simulink library "GoodWe_lib"  (Simulink 3.00)
libraries: mathlib x2, inoutlib x1
settings Model: MaskType=REX sequence  MaskIconFrame=on  MaskIconOpaque=on  MaskIconRotate=none  MaskIconUnits=autoscale

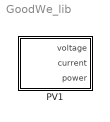
== system GoodWe_lib ==
  PV1 : Subsystem  mask(REX sequence){id=1}
      mask prompts: id "String ID"

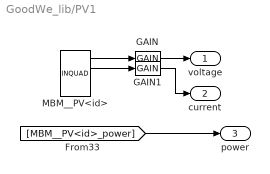
== system GoodWe_lib/PV1 ==
  GAIN : mathlib/GAIN  k=0.1
  GAIN1 : mathlib/GAIN  k=0.1
  MBM__PV<id> : inoutlib/INQUAD
  voltage : Outport  Port=1  OutDataTypeStr=Inherit: auto
  current : Outport  Port=2  OutDataTypeStr=Inherit: auto
  power : Outport  Port=3  OutDataTypeStr=Inherit: auto
  wires:
  [MBM__PV<id>_power] -> power/1
  GAIN/1 -> voltage/1
  GAIN1/1 -> current/1
  MBM__PV<id>/1 -> GAIN/1
  MBM__PV<id>/2 -> GAIN1/1
